simulink model "myfuzzy"  (R2017a)
settings: Solver=VariableStepAuto  StartTime=0.0  StopTime=10.0  RelTol=0.001
undefined symbols (not defined in the file or in its folder): f1
libraries: fuzblock x1
settings Model: Creator=Administrator  LastModifiedBy=Lenovo
settings SolverCC: ZeroCrossControl=DisableAll  ZeroCrossAlgorithm=Adaptive

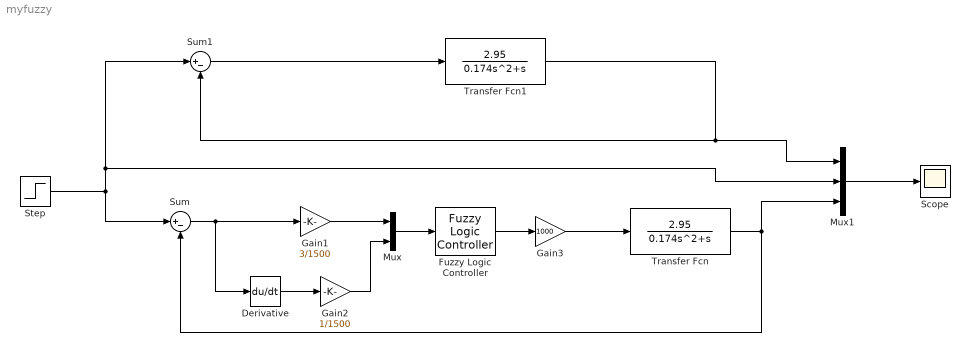
== system myfuzzy ==
  Derivative : Derivative
  Fuzzy Logic Controller : fuzblock/Fuzzy Logic  Controller  fis=[f1]
  Gain1 : Gain  Gain=3/1500
  Gain2 : Gain  Gain=1/1500
  Gain3 : Gain  Gain=1000
  Mux : Mux  Inputs=2
  Mux1 : Mux  Inputs=3
  Scope : Scope
  Step : Step  After=1500  SampleTime=0.01
  Sum : Sum  Inputs=|+-
  Sum1 : Sum  Inputs=|+-
  Transfer Fcn : TransferFcn  Numerator=[2.95]  Denominator=[0.174 1 0]
  Transfer Fcn1 : TransferFcn  Numerator=[2.95]  Denominator=[0.174 1 0]
  wires:
  Sum/1 -> Derivative/1, Gain1/1
  Derivative/1 -> Gain2/1
  Step/1 -> Mux1/2, Sum1/1, Sum/1
  Sum1/1 -> Transfer Fcn1/1
  Mux1/1 -> Scope/1
  Transfer Fcn1/1 -> Mux1/1, Sum1/2
  Transfer Fcn/1 -> Mux1/3, Sum/2
  Gain1/1 -> Mux/1
  Gain2/1 -> Mux/2
  Gain3/1 -> Transfer Fcn/1
  Mux/1 -> Fuzzy Logic Controller/1
  Fuzzy Logic Controller/1 -> Gain3/1
